simulink model "gm_uz_pmsm_model_9ph_working"  (R2021a)
settings: Solver=FixedStepAuto  StartTime=0.0  StopTime=0.04  RelTol=1e-3
PreLoadFcn:
  | uz_pmsm_model_9ph_init_parameter
undefined symbols (not defined in the file or in its folder): a, b, c, friction_coefficient, inertia, k_i_d, k_p_d, k_p_q, L_d, L_o1, L_o2, L_q, L_x1, L_x2, L_y1, L_y2, L_zero, polepair, psi_pm, R_1, static_friction_torque
libraries: hdlmdlgenlib x182, hdlsllib x90, simulink x3, pid_lib x2
(part 3 of 4)

== system gm_uz_pmsm_model_9ph_working/uz_pmsm_model_9ph/Data Type Conversion18 ==
  In1 : Inport
  Data Type Conversion18 : DataTypeConversion  OutDataTypeStr=single  RndMeth=Nearest  SampleTime=2e-09
  Data Type Conversion18_pd1 : Delay  DelayLength=3
  Out1 : Outport
  wires:
  In1/1 -> Data Type Conversion18/1
  Data Type Conversion18/1 -> Data Type Conversion18_pd1/1
  Data Type Conversion18_pd1/1 -> Out1/1

== system gm_uz_pmsm_model_9ph_working/uz_pmsm_model_9ph/Data Type Conversion19 ==
  In1 : Inport
  Data Type Conversion19 : DataTypeConversion  OutDataTypeStr=single  RndMeth=Nearest  SampleTime=2e-09
  Data Type Conversion19_pd1 : Delay  DelayLength=3
  Out1 : Outport
  wires:
  In1/1 -> Data Type Conversion19/1
  Data Type Conversion19/1 -> Data Type Conversion19_pd1/1
  Data Type Conversion19_pd1/1 -> Out1/1

== system gm_uz_pmsm_model_9ph_working/uz_pmsm_model_9ph/Data Type Conversion20 ==
  In1 : Inport
  Data Type Conversion20 : DataTypeConversion  OutDataTypeStr=single  RndMeth=Nearest  SampleTime=2e-09
  Data Type Conversion20_pd1 : Delay  DelayLength=3
  Out1 : Outport
  wires:
  In1/1 -> Data Type Conversion20/1
  Data Type Conversion20/1 -> Data Type Conversion20_pd1/1
  Data Type Conversion20_pd1/1 -> Out1/1

== system gm_uz_pmsm_model_9ph_working/uz_pmsm_model_9ph/Data Type Conversion21 ==
  In1 : Inport
  Data Type Conversion21 : DataTypeConversion  OutDataTypeStr=double  RndMeth=Nearest  SampleTime=2e-09
  Data Type Conversion21_pd1 : Delay  DelayLength=3
  Out1 : Outport
  wires:
  In1/1 -> Data Type Conversion21/1
  Data Type Conversion21/1 -> Data Type Conversion21_pd1/1
  Data Type Conversion21_pd1/1 -> Out1/1

== system gm_uz_pmsm_model_9ph_working/uz_pmsm_model_9ph/Data Type Conversion22 ==
  In1 : Inport
  Data Type Conversion22 : DataTypeConversion  OutDataTypeStr=single  RndMeth=Nearest  SampleTime=2e-09
  Data Type Conversion22_pd1 : Delay  DelayLength=6
  Out1 : Outport
  wires:
  In1/1 -> Data Type Conversion22/1
  Data Type Conversion22/1 -> Data Type Conversion22_pd1/1
  Data Type Conversion22_pd1/1 -> Out1/1

== system gm_uz_pmsm_model_9ph_working/uz_pmsm_model_9ph/Data Type Conversion221 ==
  In1 : Inport
  Data Type Conversion221 : DataTypeConversion  OutDataTypeStr=double  RndMeth=Nearest  SampleTime=2e-09
  Data Type Conversion221_pd1 : Delay  DelayLength=3
  Out1 : Outport
  wires:
  In1/1 -> Data Type Conversion221/1
  Data Type Conversion221/1 -> Data Type Conversion221_pd1/1
  Data Type Conversion221_pd1/1 -> Out1/1

== system gm_uz_pmsm_model_9ph_working/uz_pmsm_model_9ph/Data Type Conversion23 ==
  In1 : Inport
  Data Type Conversion23 : DataTypeConversion  OutDataTypeStr=single  RndMeth=Nearest  SampleTime=2e-09
  Data Type Conversion23_pd1 : Delay  DelayLength=3
  Out1 : Outport
  wires:
  In1/1 -> Data Type Conversion23/1
  Data Type Conversion23/1 -> Data Type Conversion23_pd1/1
  Data Type Conversion23_pd1/1 -> Out1/1

== system gm_uz_pmsm_model_9ph_working/uz_pmsm_model_9ph/Data Type Conversion24 ==
  In1 : Inport
  Data Type Conversion24 : DataTypeConversion  OutDataTypeStr=double  RndMeth=Nearest  SampleTime=2e-09
  Data Type Conversion24_pd1 : Delay  DelayLength=3
  Out1 : Outport
  wires:
  In1/1 -> Data Type Conversion24/1
  Data Type Conversion24/1 -> Data Type Conversion24_pd1/1
  Data Type Conversion24_pd1/1 -> Out1/1

== system gm_uz_pmsm_model_9ph_working/uz_pmsm_model_9ph/Data Type Conversion25 ==
  In1 : Inport
  Data Type Conversion25 : DataTypeConversion  OutDataTypeStr=double  RndMeth=Nearest  SampleTime=2e-09
  Data Type Conversion25_pd1 : Delay  DelayLength=3
  Out1 : Outport
  wires:
  In1/1 -> Data Type Conversion25/1
  Data Type Conversion25/1 -> Data Type Conversion25_pd1/1
  Data Type Conversion25_pd1/1 -> Out1/1

== system gm_uz_pmsm_model_9ph_working/uz_pmsm_model_9ph/Data Type Conversion26 ==
  In1 : Inport
  Data Type Conversion26 : DataTypeConversion  OutDataTypeStr=double  RndMeth=Nearest  SampleTime=2e-09
  Data Type Conversion26_pd1 : Delay  DelayLength=3
  Out1 : Outport
  wires:
  In1/1 -> Data Type Conversion26/1
  Data Type Conversion26/1 -> Data Type Conversion26_pd1/1
  Data Type Conversion26_pd1/1 -> Out1/1

== system gm_uz_pmsm_model_9ph_working/uz_pmsm_model_9ph/Data Type Conversion27 ==
  In1 : Inport
  Data Type Conversion27 : DataTypeConversion  OutDataTypeStr=double  RndMeth=Nearest  SampleTime=2e-09
  Data Type Conversion27_pd1 : Delay  DelayLength=3
  Out1 : Outport
  wires:
  In1/1 -> Data Type Conversion27/1
  Data Type Conversion27/1 -> Data Type Conversion27_pd1/1
  Data Type Conversion27_pd1/1 -> Out1/1

== system gm_uz_pmsm_model_9ph_working/uz_pmsm_model_9ph/Data Type Conversion28 ==
  In1 : Inport
  Data Type Conversion28 : DataTypeConversion  OutDataTypeStr=double  RndMeth=Nearest  SampleTime=2e-09
  Data Type Conversion28_pd1 : Delay  DelayLength=3
  Out1 : Outport
  wires:
  In1/1 -> Data Type Conversion28/1
  Data Type Conversion28/1 -> Data Type Conversion28_pd1/1
  Data Type Conversion28_pd1/1 -> Out1/1

== system gm_uz_pmsm_model_9ph_working/uz_pmsm_model_9ph/Data Type Conversion29 ==
  In1 : Inport
  Data Type Conversion29 : DataTypeConversion  OutDataTypeStr=double  RndMeth=Nearest  SampleTime=2e-09
  Data Type Conversion29_pd1 : Delay  DelayLength=3
  Out1 : Outport
  wires:
  In1/1 -> Data Type Conversion29/1
  Data Type Conversion29/1 -> Data Type Conversion29_pd1/1
  Data Type Conversion29_pd1/1 -> Out1/1

== system gm_uz_pmsm_model_9ph_working/uz_pmsm_model_9ph/Data Type Conversion30 ==
  In1 : Inport
  Data Type Conversion30 : DataTypeConversion  OutDataTypeStr=double  RndMeth=Nearest  SampleTime=2e-09
  Data Type Conversion30_pd1 : Delay  DelayLength=3
  Out1 : Outport
  wires:
  In1/1 -> Data Type Conversion30/1
  Data Type Conversion30/1 -> Data Type Conversion30_pd1/1
  Data Type Conversion30_pd1/1 -> Out1/1

== system gm_uz_pmsm_model_9ph_working/uz_pmsm_model_9ph/Data Type Conversion32 ==
  In1 : Inport
  Data Type Conversion32 : DataTypeConversion  OutDataTypeStr=single  RndMeth=Nearest  SampleTime=2e-09
  Data Type Conversion32_pd1 : Delay  DelayLength=6
  Out1 : Outport
  wires:
  In1/1 -> Data Type Conversion32/1
  Data Type Conversion32/1 -> Data Type Conversion32_pd1/1
  Data Type Conversion32_pd1/1 -> Out1/1

== system gm_uz_pmsm_model_9ph_working/uz_pmsm_model_9ph/Data Type Conversion8 ==
  In1 : Inport
  Data Type Conversion8 : DataTypeConversion  OutDataTypeStr=single  RndMeth=Nearest  SampleTime=2e-09
  Data Type Conversion8_pd1 : Delay  DelayLength=3
  Out1 : Outport
  wires:
  In1/1 -> Data Type Conversion8/1
  Data Type Conversion8/1 -> Data Type Conversion8_pd1/1
  Data Type Conversion8_pd1/1 -> Out1/1

== system gm_uz_pmsm_model_9ph_working/uz_pmsm_model_9ph/Divide ==
  In1 : Inport
  In2 : Inport  Port=2
  Divide : Product  Inputs=**  OutDataTypeStr=single  SampleTime=2e-09
  Divide_pd1 : Delay  DelayLength=6
  Out1 : Outport
  wires:
  In1/1 -> Divide/1
  In2/1 -> Divide/2
  Divide/1 -> Divide_pd1/1
  Divide_pd1/1 -> Out1/1

== system gm_uz_pmsm_model_9ph_working/uz_pmsm_model_9ph/Divide1 ==
  In1 : Inport
  In2 : Inport  Port=2
  Divide1 : Product  Inputs=**  OutDataTypeStr=single  SampleTime=2e-09
  Divide1_pd1 : Delay  DelayLength=6
  Out1 : Outport
  wires:
  In1/1 -> Divide1/1
  In2/1 -> Divide1/2
  Divide1/1 -> Divide1_pd1/1
  Divide1_pd1/1 -> Out1/1

== system gm_uz_pmsm_model_9ph_working/uz_pmsm_model_9ph/Divide10 ==
  In1 : Inport
  In2 : Inport  Port=2
  Divide10 : Product  Inputs=**  OutDataTypeStr=single  SampleTime=2e-09
  Divide10_pd1 : Delay  DelayLength=6
  Out1 : Outport
  wires:
  In1/1 -> Divide10/1
  In2/1 -> Divide10/2
  Divide10/1 -> Divide10_pd1/1
  Divide10_pd1/1 -> Out1/1

== system gm_uz_pmsm_model_9ph_working/uz_pmsm_model_9ph/Divide11 ==
  In1 : Inport
  In2 : Inport  Port=2
  Divide11 : Product  Inputs=**  OutDataTypeStr=single  SampleTime=2e-09
  Divide11_pd1 : Delay  DelayLength=6
  Out1 : Outport
  wires:
  In1/1 -> Divide11/1
  In2/1 -> Divide11/2
  Divide11/1 -> Divide11_pd1/1
  Divide11_pd1/1 -> Out1/1

== system gm_uz_pmsm_model_9ph_working/uz_pmsm_model_9ph/Divide12 ==
  In1 : Inport
  In2 : Inport  Port=2
  Divide12 : Product  Inputs=**  OutDataTypeStr=single  SampleTime=2e-09
  Divide12_pd1 : Delay  DelayLength=6
  Out1 : Outport
  wires:
  In1/1 -> Divide12/1
  In2/1 -> Divide12/2
  Divide12/1 -> Divide12_pd1/1
  Divide12_pd1/1 -> Out1/1

== system gm_uz_pmsm_model_9ph_working/uz_pmsm_model_9ph/Divide13 ==
  In1 : Inport
  In2 : Inport  Port=2
  Divide13 : Product  Inputs=**  OutDataTypeStr=single  SampleTime=2e-09
  Divide13_pd1 : Delay  DelayLength=6
  Out1 : Outport
  wires:
  In1/1 -> Divide13/1
  In2/1 -> Divide13/2
  Divide13/1 -> Divide13_pd1/1
  Divide13_pd1/1 -> Out1/1

== system gm_uz_pmsm_model_9ph_working/uz_pmsm_model_9ph/Divide2 ==
  In1 : Inport
  In2 : Inport  Port=2
  Divide2 : Product  Inputs=**  OutDataTypeStr=single  SampleTime=2e-09
  Divide2_pd1 : Delay  DelayLength=6
  Out1 : Outport
  wires:
  In1/1 -> Divide2/1
  In2/1 -> Divide2/2
  Divide2/1 -> Divide2_pd1/1
  Divide2_pd1/1 -> Out1/1

== system gm_uz_pmsm_model_9ph_working/uz_pmsm_model_9ph/Divide3 ==
  In1 : Inport
  In2 : Inport  Port=2
  Divide3 : Product  Inputs=**  OutDataTypeStr=single  SampleTime=2e-09
  Divide3_pd1 : Delay  DelayLength=6
  Out1 : Outport
  wires:
  In1/1 -> Divide3/1
  In2/1 -> Divide3/2
  Divide3/1 -> Divide3_pd1/1
  Divide3_pd1/1 -> Out1/1

== system gm_uz_pmsm_model_9ph_working/uz_pmsm_model_9ph/Divide4 ==
  In1 : Inport
  In2 : Inport  Port=2
  Divide4 : Product  Inputs=**  OutDataTypeStr=single  SampleTime=2e-09
  Divide4_pd1 : Delay  DelayLength=6
  Out1 : Outport
  wires:
  In1/1 -> Divide4/1
  In2/1 -> Divide4/2
  Divide4/1 -> Divide4_pd1/1
  Divide4_pd1/1 -> Out1/1

== system gm_uz_pmsm_model_9ph_working/uz_pmsm_model_9ph/Divide5 ==
  In1 : Inport
  In2 : Inport  Port=2
  Divide5 : Product  Inputs=**  OutDataTypeStr=single  SampleTime=2e-09
  Divide5_pd1 : Delay  DelayLength=6
  Out1 : Outport
  wires:
  In1/1 -> Divide5/1
  In2/1 -> Divide5/2
  Divide5/1 -> Divide5_pd1/1
  Divide5_pd1/1 -> Out1/1

== system gm_uz_pmsm_model_9ph_working/uz_pmsm_model_9ph/Divide6 ==
  In1 : Inport
  In2 : Inport  Port=2
  Divide6 : Product  Inputs=**  OutDataTypeStr=single  SampleTime=2e-09
  Divide6_pd1 : Delay  DelayLength=6
  Out1 : Outport
  wires:
  In1/1 -> Divide6/1
  In2/1 -> Divide6/2
  Divide6/1 -> Divide6_pd1/1
  Divide6_pd1/1 -> Out1/1

== system gm_uz_pmsm_model_9ph_working/uz_pmsm_model_9ph/Divide7 ==
  In1 : Inport
  In2 : Inport  Port=2
  Divide7 : Product  Inputs=**  OutDataTypeStr=single  SampleTime=2e-09
  Divide7_pd1 : Delay  DelayLength=6
  Out1 : Outport
  wires:
  In1/1 -> Divide7/1
  In2/1 -> Divide7/2
  Divide7/1 -> Divide7_pd1/1
  Divide7_pd1/1 -> Out1/1

== system gm_uz_pmsm_model_9ph_working/uz_pmsm_model_9ph/Divide8 ==
  In1 : Inport
  In2 : Inport  Port=2
  Divide8 : Product  Inputs=**  OutDataTypeStr=single  SampleTime=2e-09
  Divide8_pd1 : Delay  DelayLength=6
  Out1 : Outport
  wires:
  In1/1 -> Divide8/1
  In2/1 -> Divide8/2
  Divide8/1 -> Divide8_pd1/1
  Divide8_pd1/1 -> Out1/1

== system gm_uz_pmsm_model_9ph_working/uz_pmsm_model_9ph/Divide9 ==
  In1 : Inport
  In2 : Inport  Port=2
  Divide9 : Product  Inputs=**  OutDataTypeStr=single  SampleTime=2e-09
  Divide9_pd1 : Delay  DelayLength=6
  Out1 : Outport
  wires:
  In1/1 -> Divide9/1
  In2/1 -> Divide9/2
  Divide9/1 -> Divide9_pd1/1
  Divide9_pd1/1 -> Out1/1

== system gm_uz_pmsm_model_9ph_working/uz_pmsm_model_9ph/Factor ==
  In1 : Inport
  In2 : Inport  Port=2
  Factor : Product  Inputs=**  OutDataTypeStr=single  SampleTime=2e-09
  Factor_pd1 : Delay  DelayLength=6
  Out1 : Outport
  wires:
  In1/1 -> Factor/1
  In2/1 -> Factor/2
  Factor/1 -> Factor_pd1/1
  Factor_pd1/1 -> Out1/1

== system gm_uz_pmsm_model_9ph_working/uz_pmsm_model_9ph/Gain ==
  In1 : Inport
  In2 : Inport  Port=2
  Gain : Product  Inputs=**  OutDataTypeStr=double  SampleTime=2e-09
  Gain_pd1 : Delay  DelayLength=6
  Out1 : Outport
  wires:
  In1/1 -> Gain/1
  In2/1 -> Gain/2
  Gain/1 -> Gain_pd1/1
  Gain_pd1/1 -> Out1/1

== system gm_uz_pmsm_model_9ph_working/uz_pmsm_model_9ph/Gain1 ==
  In1 : Inport
  In2 : Inport  Port=2
  Gain1 : Product  Inputs=**  OutDataTypeStr=double  SampleTime=2e-09
  Gain1_pd1 : Delay  DelayLength=6
  Out1 : Outport
  wires:
  In1/1 -> Gain1/1
  In2/1 -> Gain1/2
  Gain1/1 -> Gain1_pd1/1
  Gain1_pd1/1 -> Out1/1

== system gm_uz_pmsm_model_9ph_working/uz_pmsm_model_9ph/Gain2 ==
  In1 : Inport
  In2 : Inport  Port=2
  Gain2 : Product  Inputs=**  OutDataTypeStr=double  SampleTime=2e-09
  Gain2_pd1 : Delay  DelayLength=6
  Out1 : Outport
  wires:
  In1/1 -> Gain2/1
  In2/1 -> Gain2/2
  Gain2/1 -> Gain2_pd1/1
  Gain2_pd1/1 -> Out1/1

== system gm_uz_pmsm_model_9ph_working/uz_pmsm_model_9ph/Gain3 ==
  In1 : Inport
  In2 : Inport  Port=2
  Gain3 : Product  Inputs=**  OutDataTypeStr=double  SampleTime=2e-09
  Gain3_pd1 : Delay  DelayLength=6
  Out1 : Outport
  wires:
  In1/1 -> Gain3/1
  In2/1 -> Gain3/2
  Gain3/1 -> Gain3_pd1/1
  Gain3_pd1/1 -> Out1/1

== system gm_uz_pmsm_model_9ph_working/uz_pmsm_model_9ph/Gain4 ==
  In1 : Inport
  In2 : Inport  Port=2
  Gain4 : Product  Inputs=**  OutDataTypeStr=double  SampleTime=2e-09
  Gain4_pd1 : Delay  DelayLength=6
  Out1 : Outport
  wires:
  In1/1 -> Gain4/1
  In2/1 -> Gain4/2
  Gain4/1 -> Gain4_pd1/1
  Gain4_pd1/1 -> Out1/1

== system gm_uz_pmsm_model_9ph_working/uz_pmsm_model_9ph/Gain5 ==
  In1 : Inport
  In2 : Inport  Port=2
  Gain5 : Product  Inputs=**  OutDataTypeStr=double  SampleTime=2e-09
  Gain5_pd1 : Delay  DelayLength=6
  Out1 : Outport
  wires:
  In1/1 -> Gain5/1
  In2/1 -> Gain5/2
  Gain5/1 -> Gain5_pd1/1
  Gain5_pd1/1 -> Out1/1

== system gm_uz_pmsm_model_9ph_working/uz_pmsm_model_9ph/Gain6 ==
  In1 : Inport
  In2 : Inport  Port=2
  Gain6 : Product  Inputs=**  OutDataTypeStr=double  SampleTime=2e-09
  Gain6_pd1 : Delay  DelayLength=6
  Out1 : Outport
  wires:
  In1/1 -> Gain6/1
  In2/1 -> Gain6/2
  Gain6/1 -> Gain6_pd1/1
  Gain6_pd1/1 -> Out1/1

== system gm_uz_pmsm_model_9ph_working/uz_pmsm_model_9ph/Gain7 ==
  In1 : Inport
  In2 : Inport  Port=2
  Gain7 : Product  Inputs=**  OutDataTypeStr=double  SampleTime=2e-09
  Gain7_pd1 : Delay  DelayLength=6
  Out1 : Outport
  wires:
  In1/1 -> Gain7/1
  In2/1 -> Gain7/2
  Gain7/1 -> Gain7_pd1/1
  Gain7_pd1/1 -> Out1/1

== system gm_uz_pmsm_model_9ph_working/uz_pmsm_model_9ph/Gain8 ==
  In1 : Inport
  In2 : Inport  Port=2
  Gain8 : Product  Inputs=**  OutDataTypeStr=double  SampleTime=2e-09
  Gain8_pd1 : Delay  DelayLength=6
  Out1 : Outport
  wires:
  In1/1 -> Gain8/1
  In2/1 -> Gain8/2
  Gain8/1 -> Gain8_pd1/1
  Gain8_pd1/1 -> Out1/1

== system gm_uz_pmsm_model_9ph_working/uz_pmsm_model_9ph/Gain9 ==
  In1 : Inport
  In2 : Inport  Port=2
  Gain9 : Product  Inputs=**  OutDataTypeStr=double  SampleTime=2e-09
  Gain9_pd1 : Delay  DelayLength=6
  Out1 : Outport
  wires:
  In1/1 -> Gain9/1
  In2/1 -> Gain9/2
  Gain9/1 -> Gain9_pd1/1
  Gain9_pd1/1 -> Out1/1

== system gm_uz_pmsm_model_9ph_working/uz_pmsm_model_9ph/Product ==
  In1 : Inport
  In2 : Inport  Port=2
  Product : Product  Inputs=**  OutDataTypeStr=single  SampleTime=2e-09
  Product_pd1 : Delay  DelayLength=6
  Out1 : Outport
  wires:
  In1/1 -> Product/1
  In2/1 -> Product/2
  Product/1 -> Product_pd1/1
  Product_pd1/1 -> Out1/1

== system gm_uz_pmsm_model_9ph_working/uz_pmsm_model_9ph/Product1 ==
  In1 : Inport
  In2 : Inport  Port=2
  Product1 : Product  Inputs=**  OutDataTypeStr=single  SampleTime=2e-09
  Product1_pd1 : Delay  DelayLength=6
  Out1 : Outport
  wires:
  In1/1 -> Product1/1
  In2/1 -> Product1/2
  Product1/1 -> Product1_pd1/1
  Product1_pd1/1 -> Out1/1

== system gm_uz_pmsm_model_9ph_working/uz_pmsm_model_9ph/Product10 ==
  In1 : Inport
  In2 : Inport  Port=2
  Product10 : Product  Inputs=**  OutDataTypeStr=single  SampleTime=2e-09
  Product10_pd1 : Delay  DelayLength=6
  Out1 : Outport
  wires:
  In1/1 -> Product10/1
  In2/1 -> Product10/2
  Product10/1 -> Product10_pd1/1
  Product10_pd1/1 -> Out1/1

== system gm_uz_pmsm_model_9ph_working/uz_pmsm_model_9ph/Product11 ==
  In1 : Inport
  In2 : Inport  Port=2
  Product11 : Product  Inputs=**  OutDataTypeStr=single  SampleTime=2e-09
  Product11_pd1 : Delay  DelayLength=6
  Out1 : Outport
  wires:
  In1/1 -> Product11/1
  In2/1 -> Product11/2
  Product11/1 -> Product11_pd1/1
  Product11_pd1/1 -> Out1/1

== system gm_uz_pmsm_model_9ph_working/uz_pmsm_model_9ph/Product2 ==
  In1 : Inport
  In2 : Inport  Port=2
  Product2 : Product  Inputs=**  OutDataTypeStr=single  SampleTime=2e-09
  Product2_pd1 : Delay  DelayLength=6
  Out1 : Outport
  wires:
  In1/1 -> Product2/1
  In2/1 -> Product2/2
  Product2/1 -> Product2_pd1/1
  Product2_pd1/1 -> Out1/1

== system gm_uz_pmsm_model_9ph_working/uz_pmsm_model_9ph/Product3 ==
  In1 : Inport
  In2 : Inport  Port=2
  Product3 : Product  Inputs=**  OutDataTypeStr=single  SampleTime=2e-09
  Product3_pd1 : Delay  DelayLength=6
  Out1 : Outport
  wires:
  In1/1 -> Product3/1
  In2/1 -> Product3/2
  Product3/1 -> Product3_pd1/1
  Product3_pd1/1 -> Out1/1

== system gm_uz_pmsm_model_9ph_working/uz_pmsm_model_9ph/Product5 ==
  In1 : Inport
  In2 : Inport  Port=2
  Product5 : Product  Inputs=**  OutDataTypeStr=single  SampleTime=2e-09
  Product5_pd1 : Delay  DelayLength=6
  Out1 : Outport
  wires:
  In1/1 -> Product5/1
  In2/1 -> Product5/2
  Product5/1 -> Product5_pd1/1
  Product5_pd1/1 -> Out1/1

== system gm_uz_pmsm_model_9ph_working/uz_pmsm_model_9ph/Product6 ==
  In1 : Inport
  In2 : Inport  Port=2
  Product6 : Product  Inputs=**  OutDataTypeStr=single  SampleTime=2e-09
  Product6_pd1 : Delay  DelayLength=6
  Out1 : Outport
  wires:
  In1/1 -> Product6/1
  In2/1 -> Product6/2
  Product6/1 -> Product6_pd1/1
  Product6_pd1/1 -> Out1/1

== system gm_uz_pmsm_model_9ph_working/uz_pmsm_model_9ph/Product7 ==
  In1 : Inport
  In2 : Inport  Port=2
  Product7 : Product  Inputs=**  OutDataTypeStr=single  SampleTime=2e-09
  Product7_pd1 : Delay  DelayLength=6
  Out1 : Outport
  wires:
  In1/1 -> Product7/1
  In2/1 -> Product7/2
  Product7/1 -> Product7_pd1/1
  Product7_pd1/1 -> Out1/1

== system gm_uz_pmsm_model_9ph_working/uz_pmsm_model_9ph/Product8 ==
  In1 : Inport
  In2 : Inport  Port=2
  Product8 : Product  Inputs=**  OutDataTypeStr=single  SampleTime=2e-09
  Product8_pd1 : Delay  DelayLength=6
  Out1 : Outport
  wires:
  In1/1 -> Product8/1
  In2/1 -> Product8/2
  Product8/1 -> Product8_pd1/1
  Product8_pd1/1 -> Out1/1

== system gm_uz_pmsm_model_9ph_working/uz_pmsm_model_9ph/Product9 ==
  In1 : Inport
  In2 : Inport  Port=2
  Product9 : Product  Inputs=**  OutDataTypeStr=single  SampleTime=2e-09
  Product9_pd1 : Delay  DelayLength=6
  Out1 : Outport
  wires:
  In1/1 -> Product9/1
  In2/1 -> Product9/2
  Product9/1 -> Product9_pd1/1
  Product9_pd1/1 -> Out1/1

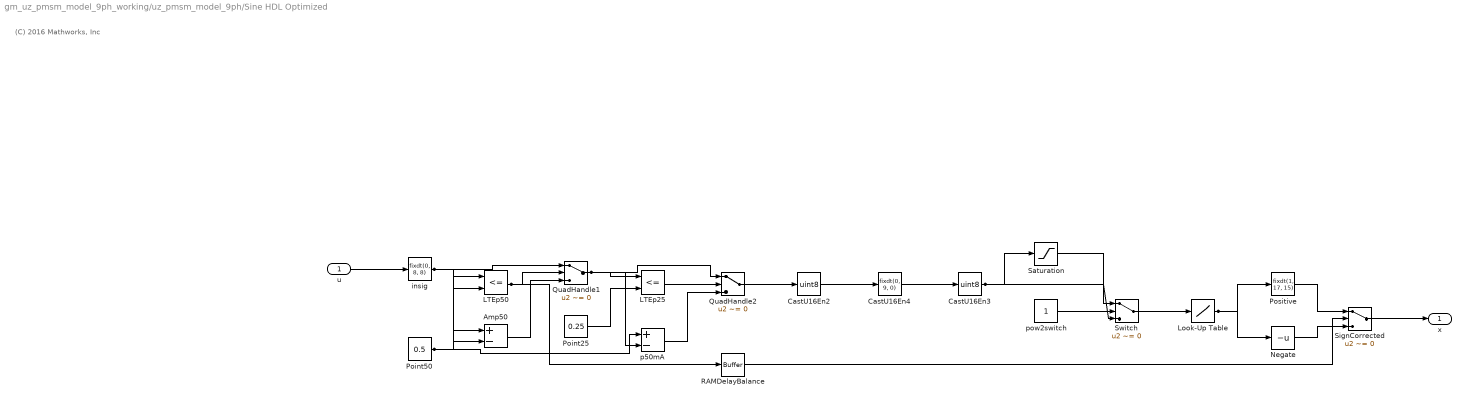
== system gm_uz_pmsm_model_9ph_working/uz_pmsm_model_9ph/Sine HDL Optimized ==
  note: (C) 2016 Mathworks, Inc
  u : Inport  OutDataTypeStr=fixdt(1, 25, 12)  SampleTime=2e-09
  Amp50 : Sum  Inputs=+-  AccumDataTypeStr=fixdt(1, 18, 17)  OutDataTypeStr=fixdt(1, 18, 17)  SampleTime=2e-09
  CastU16En2 : DataTypeConversion  OutDataTypeStr=uint8  ConvertRealWorld=Stored Integer (SI)  SampleTime=2e-09
  CastU16En3 : DataTypeConversion  OutDataTypeStr=uint8  ConvertRealWorld=Stored Integer (SI)  SampleTime=2e-09  SaturateOnIntegerOverflow=on
  CastU16En4 : DataTypeConversion  OutDataTypeStr=fixdt(0, 9, 0)  SampleTime=2e-09
  LTEp25 : RelationalOperator  Operator=<=  OutDataTypeStr=boolean  SampleTime=2e-09  RndMeth=Nearest
  LTEp50 : RelationalOperator  Operator=<=  OutDataTypeStr=boolean  SampleTime=2e-09  RndMeth=Nearest
  Look-Up Table : Lookup_n-D  NumberOfTableDimensions=1  BreakpointsForDimension1="fi(\"numerictype\",numerictype(0,8,0),\"fimath\",fimath(\"RoundingMethod\", \"Floor\",\"OverflowAction\", \"Wrap\",\"ProductMode\",\"FullPrecision\",\"SumMode\",\"FullPrecision\"),\"Value\",\"[0 1 2 3 4 5 6 7 8 9 10 11 12 13 14 15 16 17 18 19 20 21 22 23 24 25 26 27 28 29 30 31 32 33 34 35 36 37 38 39 40 41 42 43 44 45 46 47 48 49 50 51 52 53 54 55 56 57 58 59 60 61 62 63]\")"  Table="reshape(fi(\"numerictype\",numerictype(1,17,15),\"fimath\",fimath(\"RoundingMethod\", \"Floor\",\"OverflowAction\", \"Wrap\",\"ProductMode\",\"FullPrecision\",\"SumMode\",\"FullPrecision\"),\"Value\",\"[0;0.0245361328125;0.049072265625;0.073577880859375;0.0980224609375;0.122406005859375;0.146728515625;0.17095947265625;0.195098876953125;0.2191162109375;0.24298095703125;0.2667236328125;0.290283203125;0.313690185546875;0.336883544921875;0.359893798828125;0.3826904296875;0.405242919921875;0.42755126953125;0.449615478515625;0.471405029296875;0.492889404296875;0.51409912109375;0.535003662109375;0.555572509765625;0.5758056640625;0.595703125;0.615234375;0.6343994140625;0.653167724609375;0.67156982421875;0.689544677734375;0.70709228515625;0.7242431640625;0.740936279296875;0.7572021484375;0.77301025390625;0.788360595703125;0.80322265625;0.817596435546875;0.83148193359375;0.8448486328125;0.85772705078125;0.870086669921875;0.881927490234375;0.893218994140625;0.90399169921875;0.914215087890625;0.92388916015625;0.9329833984375;0.941558837890625;0.94952392578125;0.956939697265625;0.963775634765625;0.97003173828125;0.9757080078125;0.98077392578125;0.98529052734375;0.989166259765625;0.99249267578125;0.99517822265625;0.997283935546875;0.998809814453125;0.99969482421875]\"), [1  64])"  InterpMethod=Flat  ExtrapMethod=Clip  DiagnosticForOutOfRangeInput=Error  SampleTime=2e-09  OutDataTypeStr=fixdt(1, 17, 15)  InputSameDT=on
  Negate : UnaryMinus  SampleTime=2e-09
  Point25 : Constant  Value=0.25  OutDataTypeStr=fixdt(0, 17, 17)  SampleTime=2e-09
  Point50 : Constant  Value=0.5  OutDataTypeStr=fixdt(0, 17, 17)  SampleTime=2e-09
  Positive : DataTypeConversion  OutDataTypeStr=fixdt(1, 17, 15)  SampleTime=2e-09
  QuadHandle1 : Switch  Criteria=u2 ~= 0  Threshold=double(0)  OutDataTypeStr=fixdt(1, 18, 17)  SampleTime=2e-09
  QuadHandle2 : Switch  Criteria=u2 ~= 0  Threshold=double(0)  OutDataTypeStr=fixdt(0, 8, 8)  SampleTime=2e-09
  RAMDelayBalance : hdlmdlgenlib/Buffer
      settings: SourceProductBaseCode=SL
  Saturation : Saturate  UpperLimit="fi(0,0,8,0,\"hex\",\"3f\")"  LowerLimit="fi(0,0,8,0,\"hex\",\"00\")"  SampleTime=2e-09  OutDataTypeStr=uint8
  SignCorrected : Switch  Criteria=u2 ~= 0  Threshold=double(0)  OutDataTypeStr=fixdt(1, 17, 15)  SampleTime=2e-09
  Switch : Switch  Criteria=u2 ~= 0  Threshold=double(0)  OutDataTypeStr=uint8  SampleTime=2e-09
  insig : DataTypeConversion  OutDataTypeStr=fixdt(0, 8, 8)  SampleTime=2e-09
  p50mA : Sum  Inputs=+-  AccumDataTypeStr=fixdt(1, 19, 17)  OutDataTypeStr=fixdt(1, 19, 17)  SampleTime=2e-09
  pow2switch : Constant  OutDataTypeStr=boolean  SampleTime=2e-09
  x : Outport  SampleTime=2e-09
  wires:
  Amp50/1 -> QuadHandle1/3
  CastU16En2/1 -> CastU16En4/1
  CastU16En3/1 -> Switch/3, Saturation/1
  CastU16En4/1 -> CastU16En3/1
  LTEp25/1 -> QuadHandle2/2
  LTEp50/1 -> QuadHandle1/2, RAMDelayBalance/1
  Look-Up Table/1 -> Positive/1, Negate/1
  Negate/1 -> SignCorrected/3
  Point25/1 -> LTEp25/2
  Point50/1 -> p50mA/1, LTEp50/2, Amp50/2
  Positive/1 -> SignCorrected/1
  QuadHandle1/1 -> p50mA/2, QuadHandle2/1, LTEp25/1
  QuadHandle2/1 -> CastU16En2/1
  RAMDelayBalance/1 -> SignCorrected/2
  Saturation/1 -> Switch/1
  SignCorrected/1 -> x/1
  Switch/1 -> Look-Up Table/1
  insig/1 -> QuadHandle1/1, LTEp50/1, Amp50/1
  p50mA/1 -> QuadHandle2/3
  pow2switch/1 -> Switch/2
  u/1 -> insig/1

== system gm_uz_pmsm_model_9ph_working/uz_pmsm_model_9ph/Sum1 ==
  In1 : Inport
  In2 : Inport  Port=2
  Sum1 : Sum  Inputs=+-  OutDataTypeStr=single  SampleTime=2e-09
  Sum1_pd1 : Delay  DelayLength=6
  Out1 : Outport
  wires:
  In1/1 -> Sum1/1
  In2/1 -> Sum1/2
  Sum1/1 -> Sum1_pd1/1
  Sum1_pd1/1 -> Out1/1

== system gm_uz_pmsm_model_9ph_working/uz_pmsm_model_9ph/Sum1_stage2 ==
  In1 : Inport
  In2 : Inport  Port=2
  Sum1_stage2 : Sum  Inputs=+-  OutDataTypeStr=single  SampleTime=2e-09
  Sum1_stage2_pd1 : Delay  DelayLength=6
  Out1 : Outport
  wires:
  In1/1 -> Sum1_stage2/1
  In2/1 -> Sum1_stage2/2
  Sum1_stage2/1 -> Sum1_stage2_pd1/1
  Sum1_stage2_pd1/1 -> Out1/1

== system gm_uz_pmsm_model_9ph_working/uz_pmsm_model_9ph/Sum1_stage3 ==
  In1 : Inport
  In2 : Inport  Port=2
  Sum1_stage3 : Sum  Inputs=+-  OutDataTypeStr=single  SampleTime=2e-09
  Sum1_stage3_pd1 : Delay  DelayLength=6
  Out1 : Outport
  wires:
  In1/1 -> Sum1_stage3/1
  In2/1 -> Sum1_stage3/2
  Sum1_stage3/1 -> Sum1_stage3_pd1/1
  Sum1_stage3_pd1/1 -> Out1/1

== system gm_uz_pmsm_model_9ph_working/uz_pmsm_model_9ph/Sum2 ==
  In1 : Inport
  In2 : Inport  Port=2
  Sum2 : Sum  Inputs=+-  OutDataTypeStr=single  SampleTime=2e-09
  Sum2_pd1 : Delay  DelayLength=6
  Out1 : Outport
  wires:
  In1/1 -> Sum2/1
  In2/1 -> Sum2/2
  Sum2/1 -> Sum2_pd1/1
  Sum2_pd1/1 -> Out1/1

== system gm_uz_pmsm_model_9ph_working/uz_pmsm_model_9ph/Sum3 ==
  In1 : Inport
  In2 : Inport  Port=2
  Sum3 : Sum  OutDataTypeStr=double  SampleTime=2e-09
  Sum3_pd1 : Delay  DelayLength=6
  Out1 : Outport
  wires:
  In1/1 -> Sum3/1
  In2/1 -> Sum3/2
  Sum3/1 -> Sum3_pd1/1
  Sum3_pd1/1 -> Out1/1

== system gm_uz_pmsm_model_9ph_working/uz_pmsm_model_9ph/Sum31 ==
  In1 : Inport
  In2 : Inport  Port=2
  Sum31 : Sum  OutDataTypeStr=double  SampleTime=2e-09
  Sum31_pd1 : Delay  DelayLength=6
  Out1 : Outport
  wires:
  In1/1 -> Sum31/1
  In2/1 -> Sum31/2
  Sum31/1 -> Sum31_pd1/1
  Sum31_pd1/1 -> Out1/1

== system gm_uz_pmsm_model_9ph_working/uz_pmsm_model_9ph/Sum310 ==
  In1 : Inport
  In2 : Inport  Port=2
  Sum310 : Sum  OutDataTypeStr=double  SampleTime=2e-09
  Sum310_pd1 : Delay  DelayLength=6
  Out1 : Outport
  wires:
  In1/1 -> Sum310/1
  In2/1 -> Sum310/2
  Sum310/1 -> Sum310_pd1/1
  Sum310_pd1/1 -> Out1/1

== system gm_uz_pmsm_model_9ph_working/uz_pmsm_model_9ph/Sum32 ==
  In1 : Inport
  In2 : Inport  Port=2
  Sum32 : Sum  OutDataTypeStr=double  SampleTime=2e-09
  Sum32_pd1 : Delay  DelayLength=6
  Out1 : Outport
  wires:
  In1/1 -> Sum32/1
  In2/1 -> Sum32/2
  Sum32/1 -> Sum32_pd1/1
  Sum32_pd1/1 -> Out1/1

== system gm_uz_pmsm_model_9ph_working/uz_pmsm_model_9ph/Sum33 ==
  In1 : Inport
  In2 : Inport  Port=2
  Sum33 : Sum  Inputs=+-  OutDataTypeStr=single  SampleTime=2e-09
  Sum33_pd1 : Delay  DelayLength=6
  Out1 : Outport
  wires:
  In1/1 -> Sum33/1
  In2/1 -> Sum33/2
  Sum33/1 -> Sum33_pd1/1
  Sum33_pd1/1 -> Out1/1

== system gm_uz_pmsm_model_9ph_working/uz_pmsm_model_9ph/Sum34 ==
  In1 : Inport
  In2 : Inport  Port=2
  Sum34 : Sum  OutDataTypeStr=double  SampleTime=2e-09
  Sum34_pd1 : Delay  DelayLength=6
  Out1 : Outport
  wires:
  In1/1 -> Sum34/1
  In2/1 -> Sum34/2
  Sum34/1 -> Sum34_pd1/1
  Sum34_pd1/1 -> Out1/1

== system gm_uz_pmsm_model_9ph_working/uz_pmsm_model_9ph/Sum35 ==
  In1 : Inport
  In2 : Inport  Port=2
  Sum35 : Sum  OutDataTypeStr=double  SampleTime=2e-09
  Sum35_pd1 : Delay  DelayLength=6
  Out1 : Outport
  wires:
  In1/1 -> Sum35/1
  In2/1 -> Sum35/2
  Sum35/1 -> Sum35_pd1/1
  Sum35_pd1/1 -> Out1/1

== system gm_uz_pmsm_model_9ph_working/uz_pmsm_model_9ph/Sum36 ==
  In1 : Inport
  In2 : Inport  Port=2
  Sum36 : Sum  OutDataTypeStr=double  SampleTime=2e-09
  Sum36_pd1 : Delay  DelayLength=6
  Out1 : Outport
  wires:
  In1/1 -> Sum36/1
  In2/1 -> Sum36/2
  Sum36/1 -> Sum36_pd1/1
  Sum36_pd1/1 -> Out1/1

== system gm_uz_pmsm_model_9ph_working/uz_pmsm_model_9ph/Sum37 ==
  In1 : Inport
  In2 : Inport  Port=2
  Sum37 : Sum  OutDataTypeStr=double  SampleTime=2e-09
  Sum37_pd1 : Delay  DelayLength=6
  Out1 : Outport
  wires:
  In1/1 -> Sum37/1
  In2/1 -> Sum37/2
  Sum37/1 -> Sum37_pd1/1
  Sum37_pd1/1 -> Out1/1

== system gm_uz_pmsm_model_9ph_working/uz_pmsm_model_9ph/Sum38 ==
  In1 : Inport
  In2 : Inport  Port=2
  Sum38 : Sum  OutDataTypeStr=double  SampleTime=2e-09
  Sum38_pd1 : Delay  DelayLength=6
  Out1 : Outport
  wires:
  In1/1 -> Sum38/1
  In2/1 -> Sum38/2
  Sum38/1 -> Sum38_pd1/1
  Sum38_pd1/1 -> Out1/1

== system gm_uz_pmsm_model_9ph_working/uz_pmsm_model_9ph/Sum39 ==
  In1 : Inport
  In2 : Inport  Port=2
  Sum39 : Sum  OutDataTypeStr=double  SampleTime=2e-09
  Sum39_pd1 : Delay  DelayLength=6
  Out1 : Outport
  wires:
  In1/1 -> Sum39/1
  In2/1 -> Sum39/2
  Sum39/1 -> Sum39_pd1/1
  Sum39_pd1/1 -> Out1/1

== system gm_uz_pmsm_model_9ph_working/uz_pmsm_model_9ph/Sum_stage2 ==
  In1 : Inport
  In2 : Inport  Port=2
  Sum_stage2 : Sum  Inputs=+-  OutDataTypeStr=single  SampleTime=2e-09
  Sum_stage2_pd1 : Delay  DelayLength=6
  Out1 : Outport
  wires:
  In1/1 -> Sum_stage2/1
  In2/1 -> Sum_stage2/2
  Sum_stage2/1 -> Sum_stage2_pd1/1
  Sum_stage2_pd1/1 -> Out1/1

== system gm_uz_pmsm_model_9ph_working/uz_pmsm_model_9ph/Sum_stage3 ==
  In1 : Inport
  In2 : Inport  Port=2
  Sum_stage3 : Sum  OutDataTypeStr=single  SampleTime=2e-09
  Sum_stage3_pd1 : Delay  DelayLength=6
  Out1 : Outport
  wires:
  In1/1 -> Sum_stage3/1
  In2/1 -> Sum_stage3/2
  Sum_stage3/1 -> Sum_stage3_pd1/1
  Sum_stage3_pd1/1 -> Out1/1

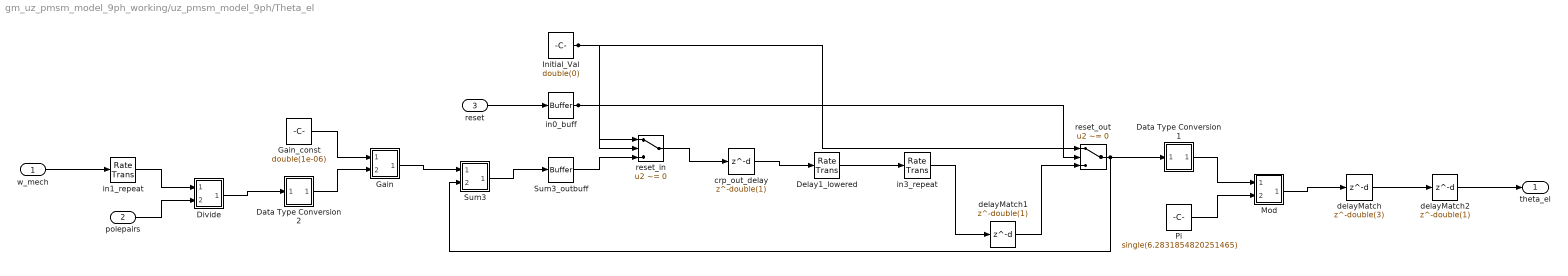
== system gm_uz_pmsm_model_9ph_working/uz_pmsm_model_9ph/Theta_el ==
  w_mech : Inport  OutDataTypeStr=single  PortDimensions=1  SampleTime=1e-06
  polepairs : Inport  Port=2  OutDataTypeStr=single  PortDimensions=1  SampleTime=2e-09
  reset : Inport  Port=3  OutDataTypeStr=boolean  PortDimensions=1  SampleTime=2e-09
  Data Type Conversion1 : Subsystem
      mask Display: disp('NFP\nconv');
  Data Type Conversion2 : Subsystem
      mask Display: disp('NFP\nconv');
  Delay1_lowered : RateTransition  OutPortSampleTimeOpt=Multiple of input port sample time  OutPortSampleTimeMultiple=500
  Divide : Subsystem
      mask Display: disp('NFP\nmul');
  Gain : Subsystem
      mask Display: disp('NFP\nmul');
  Gain_const : Constant  Value=double(1e-06)  OutDataTypeStr=double  SampleTime=2e-09
  Initial_Val : Constant  Value=double(0)  OutDataTypeStr=double  SampleTime=2e-09
  Mod : Subsystem
      mask Display: disp('NFP\nmath2');
  Pi : Constant  Value=single(6.2831854820251465)  OutDataTypeStr=single  SampleTime=2e-09
  Sum3 : Subsystem
      mask Display: disp('NFP\nadd');
  Sum3_outbuff : hdlmdlgenlib/Buffer
      settings: SourceProductBaseCode=SL
  crp_out_delay : Delay  DelayLength=double(1)  InitialCondition=0  SampleTime=2e-09
  delayMatch : Delay  DelayLength=double(3)  InitialCondition=0  SampleTime=2e-09
  delayMatch1 : Delay  DelayLength=double(1)  InitialCondition=0  SampleTime=2e-09
  delayMatch2 : Delay  DelayLength=double(1)  InitialCondition=0  SampleTime=2e-09
  in0_buff : hdlmdlgenlib/Buffer
      settings: SourceProductBaseCode=SL
  in1_repeat : RateTransition  Integrity=off  Deterministic=off  OutPortSampleTimeOpt=Multiple of input port sample time  OutPortSampleTimeMultiple=1/500
  in3_repeat : RateTransition  Integrity=off  Deterministic=off  OutPortSampleTimeOpt=Multiple of input port sample time  OutPortSampleTimeMultiple=1/500
  reset_in : Switch  Criteria=u2 ~= 0  Threshold=double(0)  OutDataTypeStr=double  SampleTime=2e-09
  reset_out : Switch  Criteria=u2 ~= 0  Threshold=double(0)  OutDataTypeStr=double  SampleTime=2e-09
  theta_el : Outport  SampleTime=2e-09
  wires:
  w_mech/1 -> in1_repeat/1
  polepairs/1 -> Divide/2(In2)
  reset/1 -> in0_buff/1
  Delay1_lowered/1 -> in3_repeat/1
  crp_out_delay/1 -> Delay1_lowered/1
  in1_repeat/1 -> Divide/1(In1)
  in3_repeat/1 -> delayMatch1/1
  delayMatch2/1 -> theta_el/1
  Pi/1 -> Mod/2(In2)
  Initial_Val/1 -> reset_out/1, reset_in/1
  Sum3_outbuff/1 -> reset_in/3
  reset_in/1 -> crp_out_delay/1
  Gain_const/1 -> Gain/1(In1)
  Mod/1(Out1) -> delayMatch/1
  Divide/1(Out1) -> Data Type Conversion2/1(In1)
  Data Type Conversion2/1(Out1) -> Gain/2(In2)
  Sum3/1(Out1) -> Sum3_outbuff/1
  Data Type Conversion1/1(Out1) -> Mod/1(In1)
  Gain/1(Out1) -> Sum3/1(In1)
  reset_out/1 -> Sum3/2(In2), Data Type Conversion1/1(In1)
  in0_buff/1 -> reset_out/2, reset_in/2
  delayMatch1/1 -> reset_out/3
  delayMatch/1 -> delayMatch2/1

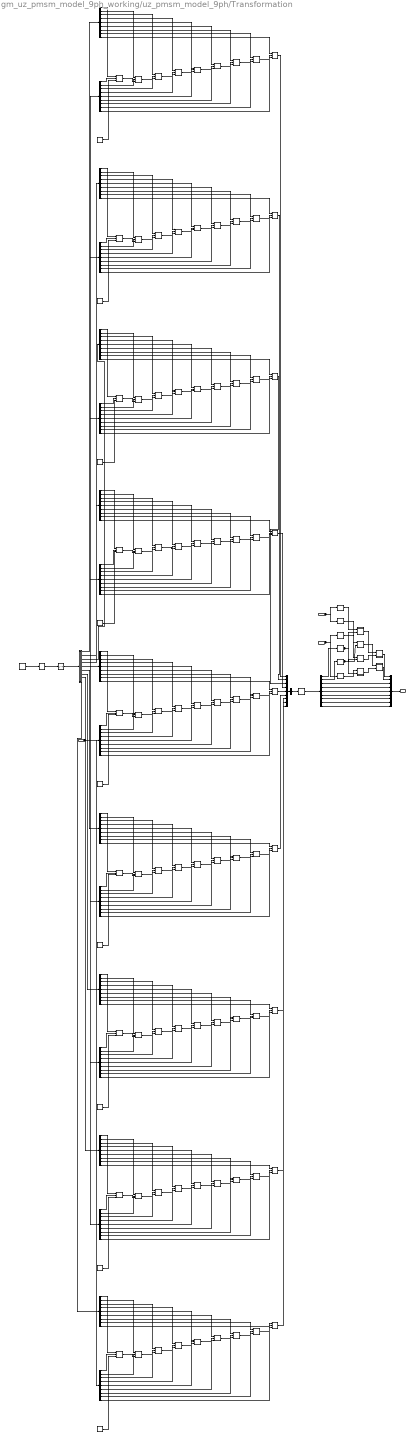
== system gm_uz_pmsm_model_9ph_working/uz_pmsm_model_9ph/Transformation ==
  in : Inport  OutDataTypeStr=fixdt(1, 25, 12)  PortDimensions=[9]  SampleTime=2e-09
  sin_theta_el : Inport  Port=2  OutDataTypeStr=single  SampleTime=2e-09
  cos_theta_el : Inport  Port=3  OutDataTypeStr=single  SampleTime=2e-09
  Add : Subsystem
      mask Display: disp('NFP\nadd');
  Add1 : Subsystem
      mask Display: disp('NFP\nadd');
  Constant1 : Constant  Value=[0.22222137451171875;0;0.22222137451171875;0;0.22222137451171875;0;0.22222137451171875;0;0.111110687255859375;-0.111110687255859375;0.1924495697021484375;0.22222137451171875;0;-0.111110687255859375;-0.1924495697021484375;-0.111110687255859375;0.1924495697021484375;0.111110687255859375;-0.111110687255859375;-0.1924495697021484375;0.22222137451171875;0;-0.111110687255859375;0.1924495697021484375;-0.111110687255859375;-0.1924495697021484375;0.111110687255859375;0.208820343017578125;0.0760040283203125;0.111110687255859375;0.1924495697021484375;-0.0385875701904296875;0.218845367431640625;-0.1702327728271484375;0.142841339111328125;-0.111110687255859375;-0.1702327728271484375;0.142841339111328125;0.111110687255859375;0.1924495697021484375;0.208820343017578125;-0.0760040283203125;-0.0385875701904296875;-0.218845367431640625;-0.111110687255859375;-0.0385875701904296875;-0.218845367431640625;0.111110687255859375;0.1924495697021484375;-0.1702327728271484375;-0.142841339111328125;0.208820343017578125;0.0760040283203125;-0.111110687255859375;0.1702327728271484375;0.142841339111328125;-0.111110687255859375;0.1924495697021484375;-0.208820343017578125;-0.0760040283203125;0.0385875701904296875;-0.218845367431640625;0.111110687255859375;-0.208820343017578125;0.0760040283203125;-0.111110687255859375;0.1924495697021484375;0.0385875701904296875;0.218845367431640625;0.1702327728271484375;0.142841339111328125;0.111110687255859375;0.0385875701904296875;-0.218845367431640625;-0.111110687255859375;0.1924495697021484375;0.1702327728271484375;-0.142841339111328125;-0.208820343017578125;0.0760040283203125;0.111110687255859375]  OutDataTypeStr=fixdt(1, 18, 19)  SampleTime=2e-09
  Data Type Conversion39 : Subsystem
      mask Display: disp('NFP\nconv');
  Data Type Conversion39_out1_0_wire : hdlmdlgenlib/Buffer
      settings: SourceProductBaseCode=SL
  Data Type Conversion39_out1_1_wire : hdlmdlgenlib/Buffer
      settings: SourceProductBaseCode=SL
  Divide : Subsystem
      mask Display: disp('NFP\nmul');
  Divide1 : Subsystem
      mask Display: disp('NFP\nmul');
  Divide2 : Subsystem
      mask Display: disp('NFP\nmul');
  Divide3 : Subsystem
      mask Display: disp('NFP\nmul');
  From{1..2,17..18} (4 alike) : hdlmdlgenlib/Buffer
      settings: SourceProductBaseCode=SL
  _adder_MultiplyAdd{,1..80} (81 alike) : hdlsllib/HDL Operations/Multiply-Add  Function=c+(a.*b)  datatype=fixdt(1, 43, 31)  DoSatur=off  FMA=off
      settings: SourceProductBaseCode=SL
  _bias{,1..8} (9 alike) : Constant  Value=double(0)  OutDataTypeStr=fixdt(1, 43, 31)  SampleTime=2e-09
  mux : Mux  Inputs=9
  t{,6..23} (19 alike) : Demux  Outputs=9
  t1 : Reshape  OutputDimensionality=Customize  OutputDimensions=[9,9]
  t2 : Math  Operator=transpose  SaturateOnIntegerOverflow=on
  t3 : Subsystem
  t4 : Mux  Inputs=9
  t5 : Concatenate  NumInputs=1  Mode=Multidimensional array  ConcatenateDimension=2
  out : Outport  SampleTime=2e-09
  wires:
  t1/1 -> t2/1
  Data Type Conversion39_out1_0_wire/1 -> Divide2/2(In2), Divide/2(In2)
  Data Type Conversion39_out1_1_wire/1 -> Divide3/2(In2), Divide1/2(In2)
  t5/1 -> Data Type Conversion39/1(In1)
  mux/1 -> out/1
  t/1 -> Data Type Conversion39_out1_0_wire/1
  t/2 -> Data Type Conversion39_out1_1_wire/1
  t/3 -> mux/3
  t/4 -> mux/4
  t/5 -> mux/5
  t/6 -> mux/6
  t/7 -> mux/7
  t/8 -> mux/8
  t/9 -> mux/9
  Constant1/1 -> t1/1
  t2/1 -> t3/1(in0)
  t3/1(out0) -> t6/1
  t3/2(out1) -> t8/1
  t3/3(out2) -> t10/1
  t3/4(out3) -> t12/1
  t3/5(out4) -> t14/1
  t3/6(out5) -> t16/1
  t3/7(out6) -> t18/1
  t3/8(out7) -> t20/1
  t3/9(out8) -> t22/1
  _adder_MultiplyAdd8/1 -> t4/1
  _adder_MultiplyAdd17/1 -> t4/2
  _adder_MultiplyAdd26/1 -> t4/3
  _adder_MultiplyAdd35/1 -> t4/4
  _adder_MultiplyAdd44/1 -> t4/5
  _adder_MultiplyAdd53/1 -> t4/6
  _adder_MultiplyAdd62/1 -> t4/7
  _adder_MultiplyAdd71/1 -> t4/8
  _adder_MultiplyAdd80/1 -> t4/9
  t4/1 -> t5/1
  _bias/1 -> _adder_MultiplyAdd/3
  t6/1 -> _adder_MultiplyAdd/1
  t7/1 -> _adder_MultiplyAdd/2
  t6/2 -> _adder_MultiplyAdd1/1
  t7/2 -> _adder_MultiplyAdd1/2
  _adder_MultiplyAdd/1 -> _adder_MultiplyAdd1/3
  t6/3 -> _adder_MultiplyAdd2/1
  t7/3 -> _adder_MultiplyAdd2/2
  _adder_MultiplyAdd1/1 -> _adder_MultiplyAdd2/3
  t6/4 -> _adder_MultiplyAdd3/1
  t7/4 -> _adder_MultiplyAdd3/2
  _adder_MultiplyAdd2/1 -> _adder_MultiplyAdd3/3
  t6/5 -> _adder_MultiplyAdd4/1
  t7/5 -> _adder_MultiplyAdd4/2
  _adder_MultiplyAdd3/1 -> _adder_MultiplyAdd4/3
  t6/6 -> _adder_MultiplyAdd5/1
  t7/6 -> _adder_MultiplyAdd5/2
  _adder_MultiplyAdd4/1 -> _adder_MultiplyAdd5/3
  t6/7 -> _adder_MultiplyAdd6/1
  t7/7 -> _adder_MultiplyAdd6/2
  _adder_MultiplyAdd5/1 -> _adder_MultiplyAdd6/3
  t6/8 -> _adder_MultiplyAdd7/1
  t7/8 -> _adder_MultiplyAdd7/2
  _adder_MultiplyAdd6/1 -> _adder_MultiplyAdd7/3
  t6/9 -> _adder_MultiplyAdd8/1
  t7/9 -> _adder_MultiplyAdd8/2
  _adder_MultiplyAdd7/1 -> _adder_MultiplyAdd8/3
  _bias1/1 -> _adder_MultiplyAdd9/3
  t8/1 -> _adder_MultiplyAdd9/1
  t9/1 -> _adder_MultiplyAdd9/2
  t8/2 -> _adder_MultiplyAdd10/1
  t9/2 -> _adder_MultiplyAdd10/2
  _adder_MultiplyAdd9/1 -> _adder_MultiplyAdd10/3
  t8/3 -> _adder_MultiplyAdd11/1
  t9/3 -> _adder_MultiplyAdd11/2
  _adder_MultiplyAdd10/1 -> _adder_MultiplyAdd11/3
  t8/4 -> _adder_MultiplyAdd12/1
  t9/4 -> _adder_MultiplyAdd12/2
  _adder_MultiplyAdd11/1 -> _adder_MultiplyAdd12/3
  t8/5 -> _adder_MultiplyAdd13/1
  t9/5 -> _adder_MultiplyAdd13/2
  _adder_MultiplyAdd12/1 -> _adder_MultiplyAdd13/3
  t8/6 -> _adder_MultiplyAdd14/1
  t9/6 -> _adder_MultiplyAdd14/2
  _adder_MultiplyAdd13/1 -> _adder_MultiplyAdd14/3
  t8/7 -> _adder_MultiplyAdd15/1
  t9/7 -> _adder_MultiplyAdd15/2
  _adder_MultiplyAdd14/1 -> _adder_MultiplyAdd15/3
  t8/8 -> _adder_MultiplyAdd16/1
  t9/8 -> _adder_MultiplyAdd16/2
  _adder_MultiplyAdd15/1 -> _adder_MultiplyAdd16/3
  t8/9 -> _adder_MultiplyAdd17/1
  t9/9 -> _adder_MultiplyAdd17/2
  _adder_MultiplyAdd16/1 -> _adder_MultiplyAdd17/3
  _bias2/1 -> _adder_MultiplyAdd18/3
  t10/1 -> _adder_MultiplyAdd18/1
  t11/1 -> _adder_MultiplyAdd18/2
  t10/2 -> _adder_MultiplyAdd19/1
  t11/2 -> _adder_MultiplyAdd19/2
  _adder_MultiplyAdd18/1 -> _adder_MultiplyAdd19/3
  t10/3 -> _adder_MultiplyAdd20/1
  t11/3 -> _adder_MultiplyAdd20/2
  _adder_MultiplyAdd19/1 -> _adder_MultiplyAdd20/3
  t10/4 -> _adder_MultiplyAdd21/1
  t11/4 -> _adder_MultiplyAdd21/2
  _adder_MultiplyAdd20/1 -> _adder_MultiplyAdd21/3
  t10/5 -> _adder_MultiplyAdd22/1
  t11/5 -> _adder_MultiplyAdd22/2
  _adder_MultiplyAdd21/1 -> _adder_MultiplyAdd22/3
  t10/6 -> _adder_MultiplyAdd23/1
  t11/6 -> _adder_MultiplyAdd23/2
  _adder_MultiplyAdd22/1 -> _adder_MultiplyAdd23/3
  t10/7 -> _adder_MultiplyAdd24/1
  t11/7 -> _adder_MultiplyAdd24/2
  _adder_MultiplyAdd23/1 -> _adder_MultiplyAdd24/3
  t10/8 -> _adder_MultiplyAdd25/1
  t11/8 -> _adder_MultiplyAdd25/2
  _adder_MultiplyAdd24/1 -> _adder_MultiplyAdd25/3
  t10/9 -> _adder_MultiplyAdd26/1
  t11/9 -> _adder_MultiplyAdd26/2
  _adder_MultiplyAdd25/1 -> _adder_MultiplyAdd26/3
  _bias3/1 -> _adder_MultiplyAdd27/3
  t12/1 -> _adder_MultiplyAdd27/1
  t13/1 -> _adder_MultiplyAdd27/2
  t12/2 -> _adder_MultiplyAdd28/1
  t13/2 -> _adder_MultiplyAdd28/2
  _adder_MultiplyAdd27/1 -> _adder_MultiplyAdd28/3
  t12/3 -> _adder_MultiplyAdd29/1
  t13/3 -> _adder_MultiplyAdd29/2
  _adder_MultiplyAdd28/1 -> _adder_MultiplyAdd29/3
  t12/4 -> _adder_MultiplyAdd30/1
  t13/4 -> _adder_MultiplyAdd30/2
  _adder_MultiplyAdd29/1 -> _adder_MultiplyAdd30/3
  t12/5 -> _adder_MultiplyAdd31/1
  t13/5 -> _adder_MultiplyAdd31/2
  _adder_MultiplyAdd30/1 -> _adder_MultiplyAdd31/3
  t12/6 -> _adder_MultiplyAdd32/1
  t13/6 -> _adder_MultiplyAdd32/2
  _adder_MultiplyAdd31/1 -> _adder_MultiplyAdd32/3
  t12/7 -> _adder_MultiplyAdd33/1
  t13/7 -> _adder_MultiplyAdd33/2
  _adder_MultiplyAdd32/1 -> _adder_MultiplyAdd33/3
  t12/8 -> _adder_MultiplyAdd34/1
  t13/8 -> _adder_MultiplyAdd34/2
  _adder_MultiplyAdd33/1 -> _adder_MultiplyAdd34/3
  t12/9 -> _adder_MultiplyAdd35/1
  t13/9 -> _adder_MultiplyAdd35/2
  _adder_MultiplyAdd34/1 -> _adder_MultiplyAdd35/3
  _bias4/1 -> _adder_MultiplyAdd36/3
  t14/1 -> _adder_MultiplyAdd36/1
  t15/1 -> _adder_MultiplyAdd36/2
  t14/2 -> _adder_MultiplyAdd37/1
  t15/2 -> _adder_MultiplyAdd37/2
  _adder_MultiplyAdd36/1 -> _adder_MultiplyAdd37/3
  t14/3 -> _adder_MultiplyAdd38/1
  t15/3 -> _adder_MultiplyAdd38/2
  _adder_MultiplyAdd37/1 -> _adder_MultiplyAdd38/3
  t14/4 -> _adder_MultiplyAdd39/1
  t15/4 -> _adder_MultiplyAdd39/2
  _adder_MultiplyAdd38/1 -> _adder_MultiplyAdd39/3
  t14/5 -> _adder_MultiplyAdd40/1
  t15/5 -> _adder_MultiplyAdd40/2
  _adder_MultiplyAdd39/1 -> _adder_MultiplyAdd40/3
  t14/6 -> _adder_MultiplyAdd41/1
  t15/6 -> _adder_MultiplyAdd41/2
  _adder_MultiplyAdd40/1 -> _adder_MultiplyAdd41/3
  t14/7 -> _adder_MultiplyAdd42/1
  t15/7 -> _adder_MultiplyAdd42/2
  _adder_MultiplyAdd41/1 -> _adder_MultiplyAdd42/3
  t14/8 -> _adder_MultiplyAdd43/1
  t15/8 -> _adder_MultiplyAdd43/2
  _adder_MultiplyAdd42/1 -> _adder_MultiplyAdd43/3
  t14/9 -> _adder_MultiplyAdd44/1
  t15/9 -> _adder_MultiplyAdd44/2
  _adder_MultiplyAdd43/1 -> _adder_MultiplyAdd44/3
  _bias5/1 -> _adder_MultiplyAdd45/3
  t16/1 -> _adder_MultiplyAdd45/1
  t17/1 -> _adder_MultiplyAdd45/2
  t16/2 -> _adder_MultiplyAdd46/1
  t17/2 -> _adder_MultiplyAdd46/2
  _adder_MultiplyAdd45/1 -> _adder_MultiplyAdd46/3
  t16/3 -> _adder_MultiplyAdd47/1
  t17/3 -> _adder_MultiplyAdd47/2
  _adder_MultiplyAdd46/1 -> _adder_MultiplyAdd47/3
  t16/4 -> _adder_MultiplyAdd48/1
  t17/4 -> _adder_MultiplyAdd48/2
  _adder_MultiplyAdd47/1 -> _adder_MultiplyAdd48/3
  t16/5 -> _adder_MultiplyAdd49/1
  t17/5 -> _adder_MultiplyAdd49/2
  _adder_MultiplyAdd48/1 -> _adder_MultiplyAdd49/3
  t16/6 -> _adder_MultiplyAdd50/1
  t17/6 -> _adder_MultiplyAdd50/2
  _adder_MultiplyAdd49/1 -> _adder_MultiplyAdd50/3
  t16/7 -> _adder_MultiplyAdd51/1
  t17/7 -> _adder_MultiplyAdd51/2
  _adder_MultiplyAdd50/1 -> _adder_MultiplyAdd51/3
  t16/8 -> _adder_MultiplyAdd52/1
  t17/8 -> _adder_MultiplyAdd52/2
  _adder_MultiplyAdd51/1 -> _adder_MultiplyAdd52/3
  t16/9 -> _adder_MultiplyAdd53/1
  t17/9 -> _adder_MultiplyAdd53/2
  _adder_MultiplyAdd52/1 -> _adder_MultiplyAdd53/3
  _bias6/1 -> _adder_MultiplyAdd54/3
  t18/1 -> _adder_MultiplyAdd54/1
  t19/1 -> _adder_MultiplyAdd54/2
  t18/2 -> _adder_MultiplyAdd55/1
  t19/2 -> _adder_MultiplyAdd55/2
  _adder_MultiplyAdd54/1 -> _adder_MultiplyAdd55/3
  t18/3 -> _adder_MultiplyAdd56/1
  t19/3 -> _adder_MultiplyAdd56/2
  _adder_MultiplyAdd55/1 -> _adder_MultiplyAdd56/3
  t18/4 -> _adder_MultiplyAdd57/1
  t19/4 -> _adder_MultiplyAdd57/2
  _adder_MultiplyAdd56/1 -> _adder_MultiplyAdd57/3
  t18/5 -> _adder_MultiplyAdd58/1
  t19/5 -> _adder_MultiplyAdd58/2
  _adder_MultiplyAdd57/1 -> _adder_MultiplyAdd58/3
  t18/6 -> _adder_MultiplyAdd59/1
  t19/6 -> _adder_MultiplyAdd59/2
  _adder_MultiplyAdd58/1 -> _adder_MultiplyAdd59/3
  t18/7 -> _adder_MultiplyAdd60/1
  t19/7 -> _adder_MultiplyAdd60/2
  _adder_MultiplyAdd59/1 -> _adder_MultiplyAdd60/3
  t18/8 -> _adder_MultiplyAdd61/1
  t19/8 -> _adder_MultiplyAdd61/2
  _adder_MultiplyAdd60/1 -> _adder_MultiplyAdd61/3
  t18/9 -> _adder_MultiplyAdd62/1
  t19/9 -> _adder_MultiplyAdd62/2
  _adder_MultiplyAdd61/1 -> _adder_MultiplyAdd62/3
  _bias7/1 -> _adder_MultiplyAdd63/3
  t20/1 -> _adder_MultiplyAdd63/1
  t21/1 -> _adder_MultiplyAdd63/2
  t20/2 -> _adder_MultiplyAdd64/1
  t21/2 -> _adder_MultiplyAdd64/2
  _adder_MultiplyAdd63/1 -> _adder_MultiplyAdd64/3
  t20/3 -> _adder_MultiplyAdd65/1
  t21/3 -> _adder_MultiplyAdd65/2
  _adder_MultiplyAdd64/1 -> _adder_MultiplyAdd65/3
  t20/4 -> _adder_MultiplyAdd66/1
  t21/4 -> _adder_MultiplyAdd66/2
  _adder_MultiplyAdd65/1 -> _adder_MultiplyAdd66/3
  t20/5 -> _adder_MultiplyAdd67/1
  t21/5 -> _adder_MultiplyAdd67/2
  _adder_MultiplyAdd66/1 -> _adder_MultiplyAdd67/3
  t20/6 -> _adder_MultiplyAdd68/1
  t21/6 -> _adder_MultiplyAdd68/2
  _adder_MultiplyAdd67/1 -> _adder_MultiplyAdd68/3
  t20/7 -> _adder_MultiplyAdd69/1
  t21/7 -> _adder_MultiplyAdd69/2
  _adder_MultiplyAdd68/1 -> _adder_MultiplyAdd69/3
  t20/8 -> _adder_MultiplyAdd70/1
  t21/8 -> _adder_MultiplyAdd70/2
  _adder_MultiplyAdd69/1 -> _adder_MultiplyAdd70/3
  t20/9 -> _adder_MultiplyAdd71/1
  t21/9 -> _adder_MultiplyAdd71/2
  _adder_MultiplyAdd70/1 -> _adder_MultiplyAdd71/3
  _bias8/1 -> _adder_MultiplyAdd72/3
  t22/1 -> _adder_MultiplyAdd72/1
  t23/1 -> _adder_MultiplyAdd72/2
  t22/2 -> _adder_MultiplyAdd73/1
  t23/2 -> _adder_MultiplyAdd73/2
  _adder_MultiplyAdd72/1 -> _adder_MultiplyAdd73/3
  t22/3 -> _adder_MultiplyAdd74/1
  t23/3 -> _adder_MultiplyAdd74/2
  _adder_MultiplyAdd73/1 -> _adder_MultiplyAdd74/3
  t22/4 -> _adder_MultiplyAdd75/1
  t23/4 -> _adder_MultiplyAdd75/2
  _adder_MultiplyAdd74/1 -> _adder_MultiplyAdd75/3
  t22/5 -> _adder_MultiplyAdd76/1
  t23/5 -> _adder_MultiplyAdd76/2
  _adder_MultiplyAdd75/1 -> _adder_MultiplyAdd76/3
  t22/6 -> _adder_MultiplyAdd77/1
  t23/6 -> _adder_MultiplyAdd77/2
  _adder_MultiplyAdd76/1 -> _adder_MultiplyAdd77/3
  t22/7 -> _adder_MultiplyAdd78/1
  t23/7 -> _adder_MultiplyAdd78/2
  _adder_MultiplyAdd77/1 -> _adder_MultiplyAdd78/3
  t22/8 -> _adder_MultiplyAdd79/1
  t23/8 -> _adder_MultiplyAdd79/2
  _adder_MultiplyAdd78/1 -> _adder_MultiplyAdd79/3
  t22/9 -> _adder_MultiplyAdd80/1
  t23/9 -> _adder_MultiplyAdd80/2
  _adder_MultiplyAdd79/1 -> _adder_MultiplyAdd80/3
  Add/1(Out1) -> mux/1
  Add1/1(Out1) -> mux/2
  Data Type Conversion39/1(Out1) -> t/1
  Divide/1(Out1) -> Add/1(In1)
  Divide1/1(Out1) -> Add/2(In2)
  Divide2/1(Out1) -> Add1/2(In2)
  Divide3/1(Out1) -> Add1/1(In1)
  From17/1 -> Divide/1(In1)
  From18/1 -> Divide1/1(In1)
  From2/1 -> Divide3/1(In1)
  From1/1 -> Divide2/1(In1)
  in/1 -> t23/1, t21/1, t19/1, t17/1, t15/1, t13/1, t11/1, t9/1, t7/1
  sin_theta_el/1 -> From18/1, From1/1
  cos_theta_el/1 -> From2/1, From17/1
